simulink model "mode06_net"  (Simulink 7.4)
settings: Solver=ode45  StartTime=0.0  StopTime=5200  RelTol=1e-3
undefined symbols (not defined in the file or in its folder): ROACH
libraries: xbsIndex_r4 x184, xps_library x20, casper_library_misc x19, dspsigops x16, casper_library_flow_control x2
(part 2 of 2)

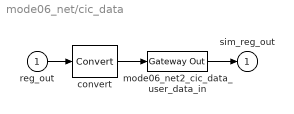
== system mode06_net/cic_data ==
  reg_out : Inport
  convert : xbsIndex_r4/Convert  arith_type=Unsigned  n_bits=32  bin_pt=0  quantization=Truncate  overflow=Wrap  latency=0  dbl_ovrd=off  pipeline=off  block_type=convert
      settings: block_version=11.4
  mode06_net2_cic_data_user_data_in : xbsIndex_r4/Gateway Out  hdl_port=on  timing_constraint=None  locs_specified=off  LOCs={}  block_type=gatewayout
      settings: infoedit="Gateway out block.  Converts Xilinx fixed point inputs into ouputs of type Simulink integer, double, or fixed point.<br><br>Hardware notes:  In hardware these blocks become top level output ports or are discarded, depending on how they are configured."  block_version=11.4
  sim_reg_out : Outport
  wires:
  mode06_net2_cic_data_user_data_in/1 -> sim_reg_out/1
  convert/1 -> mode06_net2_cic_data_user_data_in/1
  reg_out/1 -> convert/1

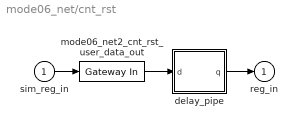
== system mode06_net/cnt_rst ==
  sim_reg_in : Inport
  delay_pipe : Subsystem
  mode06_net2_cnt_rst_user_data_out : xbsIndex_r4/Gateway In  arith_type=Unsigned  n_bits=32  bin_pt=0  quantization="Round  (unbiased: +/- Inf)"  overflow=Saturate  period=1  dbl_ovrd=off  timing_constraint=None  locs_specified=off  LOCs={}  hdl_port=on  block_type=gatewayin
      settings: infoedit="Gateway in block.  Converts inputs of type Simulink integer, double and fixed point to  Xilinx fixed point type.<br><br>Hardware notes:  In hardware these blocks become top level input ports."  block_version=11.4
  reg_in : Outport
  wires:
  delay_pipe/1(q) -> reg_in/1
  mode06_net2_cnt_rst_user_data_out/1 -> delay_pipe/1(d)
  sim_reg_in/1 -> mode06_net2_cnt_rst_user_data_out/1

== system mode06_net/dest_ip ==
  sim_reg_in : Inport
  delay_pipe : Subsystem
  mode06_net2_dest_ip_user_data_out : xbsIndex_r4/Gateway In  arith_type=Unsigned  n_bits=32  bin_pt=0  quantization="Round  (unbiased: +/- Inf)"  overflow=Saturate  period=1  dbl_ovrd=off  timing_constraint=None  locs_specified=off  LOCs={}  hdl_port=on  block_type=gatewayin
      settings: infoedit="Gateway in block.  Converts inputs of type Simulink integer, double and fixed point to  Xilinx fixed point type.<br><br>Hardware notes:  In hardware these blocks become top level input ports."  block_version=11.4
  reg_in : Outport
  wires:
  delay_pipe/1(q) -> reg_in/1
  mode06_net2_dest_ip_user_data_out/1 -> delay_pipe/1(d)
  sim_reg_in/1 -> mode06_net2_dest_ip_user_data_out/1

== system mode06_net/dest_port ==
  sim_reg_in : Inport
  delay_pipe : Subsystem
  mode06_net2_dest_port_user_data_out : xbsIndex_r4/Gateway In  arith_type=Unsigned  n_bits=32  bin_pt=0  quantization="Round  (unbiased: +/- Inf)"  overflow=Saturate  period=1  dbl_ovrd=off  timing_constraint=None  locs_specified=off  LOCs={}  hdl_port=on  block_type=gatewayin
      settings: infoedit="Gateway in block.  Converts inputs of type Simulink integer, double and fixed point to  Xilinx fixed point type.<br><br>Hardware notes:  In hardware these blocks become top level input ports."  block_version=11.4
  reg_in : Outport
  wires:
  delay_pipe/1(q) -> reg_in/1
  mode06_net2_dest_port_user_data_out/1 -> delay_pipe/1(d)
  sim_reg_in/1 -> mode06_net2_dest_port_user_data_out/1

== system mode06_net/eth_rst ==
  sim_reg_in : Inport
  delay_pipe : Subsystem
  mode06_net2_eth_rst_user_data_out : xbsIndex_r4/Gateway In  arith_type=Unsigned  n_bits=32  bin_pt=0  quantization="Round  (unbiased: +/- Inf)"  overflow=Saturate  period=1  dbl_ovrd=off  timing_constraint=None  locs_specified=off  LOCs={}  hdl_port=on  block_type=gatewayin
      settings: infoedit="Gateway in block.  Converts inputs of type Simulink integer, double and fixed point to  Xilinx fixed point type.<br><br>Hardware notes:  In hardware these blocks become top level input ports."  block_version=11.4
  reg_in : Outport
  wires:
  delay_pipe/1(q) -> reg_in/1
  mode06_net2_eth_rst_user_data_out/1 -> delay_pipe/1(d)
  sim_reg_in/1 -> mode06_net2_eth_rst_user_data_out/1

== system mode06_net/ext_sync_ctr ==
  reg_out : Inport
  convert : xbsIndex_r4/Convert  arith_type=Unsigned  n_bits=32  bin_pt=0  quantization=Truncate  overflow=Wrap  latency=0  dbl_ovrd=off  pipeline=off  block_type=convert
      settings: block_version=11.4
  mode06_net2_ext_sync_ctr_user_data_in : xbsIndex_r4/Gateway Out  hdl_port=on  timing_constraint=None  locs_specified=off  LOCs={}  block_type=gatewayout
      settings: infoedit="Gateway out block.  Converts Xilinx fixed point inputs into ouputs of type Simulink integer, double, or fixed point.<br><br>Hardware notes:  In hardware these blocks become top level output ports or are discarded, depending on how they are configured."  block_version=11.4
  sim_reg_out : Outport
  wires:
  mode06_net2_ext_sync_ctr_user_data_in/1 -> sim_reg_out/1
  convert/1 -> mode06_net2_ext_sync_ctr_user_data_in/1
  reg_out/1 -> convert/1

== system mode06_net/ip_select ==
  sim_reg_in : Inport
  delay_pipe : Subsystem
  mode06_net2_ip_select_user_data_out : xbsIndex_r4/Gateway In  arith_type=Unsigned  n_bits=32  bin_pt=0  quantization="Round  (unbiased: +/- Inf)"  overflow=Saturate  period=1  dbl_ovrd=off  timing_constraint=None  locs_specified=off  LOCs={}  hdl_port=on  block_type=gatewayin
      settings: infoedit="Gateway in block.  Converts inputs of type Simulink integer, double and fixed point to  Xilinx fixed point type.<br><br>Hardware notes:  In hardware these blocks become top level input ports."  block_version=11.4
  reg_in : Outport
  wires:
  delay_pipe/1(q) -> reg_in/1
  mode06_net2_ip_select_user_data_out/1 -> delay_pipe/1(d)
  sim_reg_in/1 -> mode06_net2_ip_select_user_data_out/1

== system mode06_net/pkt_data ==
  reg_out : Inport
  convert : xbsIndex_r4/Convert  arith_type=Unsigned  n_bits=32  bin_pt=0  quantization=Truncate  overflow=Wrap  latency=0  dbl_ovrd=off  pipeline=off  block_type=convert
      settings: block_version=11.4
  mode06_net2_pkt_data_user_data_in : xbsIndex_r4/Gateway Out  hdl_port=on  timing_constraint=None  locs_specified=off  LOCs={}  block_type=gatewayout
      settings: infoedit="Gateway out block.  Converts Xilinx fixed point inputs into ouputs of type Simulink integer, double, or fixed point.<br><br>Hardware notes:  In hardware these blocks become top level output ports or are discarded, depending on how they are configured."  block_version=11.4
  sim_reg_out : Outport
  wires:
  mode06_net2_pkt_data_user_data_in/1 -> sim_reg_out/1
  convert/1 -> mode06_net2_pkt_data_user_data_in/1
  reg_out/1 -> convert/1

== system mode06_net/port_select ==
  sim_reg_in : Inport
  delay_pipe : Subsystem
  mode06_net2_port_select_user_data_out : xbsIndex_r4/Gateway In  arith_type=Unsigned  n_bits=32  bin_pt=0  quantization="Round  (unbiased: +/- Inf)"  overflow=Saturate  period=1  dbl_ovrd=off  timing_constraint=None  locs_specified=off  LOCs={}  hdl_port=on  block_type=gatewayin
      settings: infoedit="Gateway in block.  Converts inputs of type Simulink integer, double and fixed point to  Xilinx fixed point type.<br><br>Hardware notes:  In hardware these blocks become top level input ports."  block_version=11.4
  reg_in : Outport
  wires:
  delay_pipe/1(q) -> reg_in/1
  mode06_net2_port_select_user_data_out/1 -> delay_pipe/1(d)
  sim_reg_in/1 -> mode06_net2_port_select_user_data_out/1

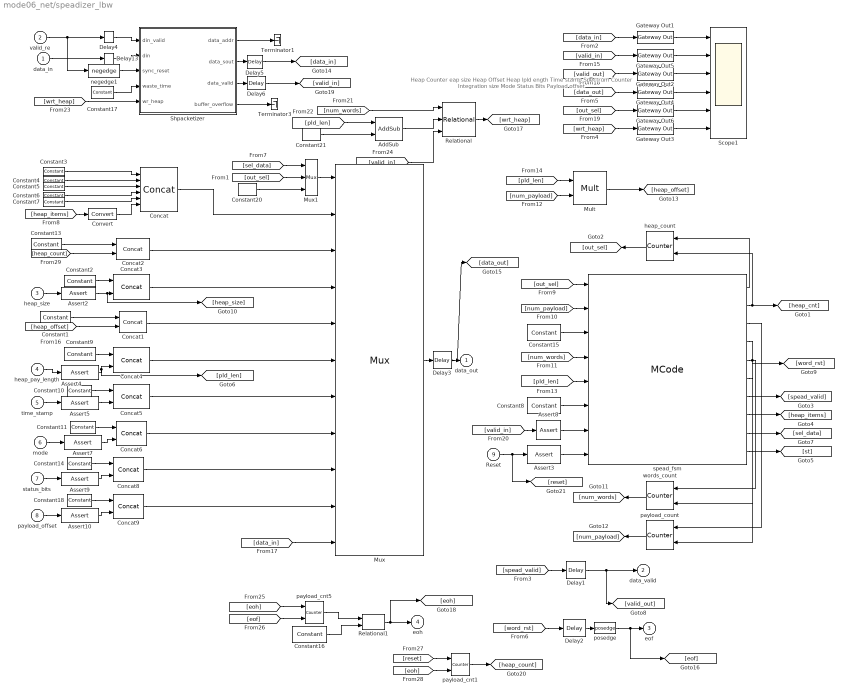
== system mode06_net/speadizer_lbw ==
  note: Heap Counter
      | eap size
      | Heap Offset
      | Heap lpld ength
      | Time stamp
      | Spectrum Counter
      | Integration size
      | Mode
      | Status Bits
      | Payload offset
  data_in : Inport
  valid_re : Inport  Port=2
  heap_size : Inport  Port=3
  heap_pay_length : Inport  Port=4
  time_stamp : Inport  Port=5
  mode : Inport  Port=6
  status_bits : Inport  Port=7
  payload_offset : Inport  Port=8
  Reset : Inport  Port=9
  AddSub : xbsIndex_r4/AddSub  mode=Subtraction  use_carryin=off  use_carryout=off  en=off  latency=0  precision=Full  arith_type=Unsigned  n_bits=16  bin_pt=14  quantization=Truncate  overflow=Wrap  dbl_ovrd=off  use_behavioral_HDL=off  hw_selection=Fabric  pipelined=off  block_type=addsub
  Assert{2,4..5,7,9..10} (6 alike) : xbsIndex_r4/Assert  assert_type=on  type_source=Explicitly  arith_type=Unsigned  n_bits=spead_lsw  bin_pt=0  assert_rate=off  rate_source=Explicitly  period=1  output_port=on  block_type=assert
      settings: block_version=11.4
  Assert3 : xbsIndex_r4/Assert  assert_type=on  type_source=Explicitly  arith_type=Boolean  n_bits=spead_lsw  bin_pt=0  assert_rate=on  rate_source=Explicitly  period=1  output_port=on  block_type=assert
      settings: block_version=11.4
  Assert8 : xbsIndex_r4/Assert  assert_type=on  type_source=Explicitly  arith_type=Boolean  n_bits=spead_lsw  bin_pt=0  assert_rate=on  rate_source=Explicitly  period=1  output_port=on  block_type=assert
      settings: block_version=11.4
  Concat : xbsIndex_r4/Concat  num_inputs=6  dbl_ovrd=off  block_type=concat
  Concat{1..6,8..9} (8 alike) : xbsIndex_r4/Concat  num_inputs=2  dbl_ovrd=off  block_type=concat
  Constant1 : xbsIndex_r4/Constant  arith_type=Unsigned  const=8388608+3  n_bits=spead_msw-spead_lsw  bin_pt=0  explicit_period=on  period=1  equ=P=C  opselect=C  inp2=PCIN>>17  opr=+  inp1=P  carry=CIN  dbl_ovrd=off  block_type=constant
      settings: block_version=11.4
  Constant10 : xbsIndex_r4/Constant  arith_type=Unsigned  const=8388608+32  n_bits=spead_msw-spead_lsw  bin_pt=0  explicit_period=on  period=1  equ=P=C  opselect=C  inp2=PCIN>>17  opr=+  inp1=P  carry=CIN  dbl_ovrd=off  block_type=constant
      settings: block_version=11.4
  Constant11 : xbsIndex_r4/Constant  arith_type=Unsigned  const=8388608+33  n_bits=spead_msw-spead_lsw  bin_pt=0  explicit_period=on  period=1  equ=P=C  opselect=C  inp2=PCIN>>17  opr=+  inp1=P  carry=CIN  dbl_ovrd=off  block_type=constant
      settings: block_version=11.4
  Constant13 : xbsIndex_r4/Constant  arith_type=Unsigned  const=8388608+1  n_bits=spead_msw-spead_lsw  bin_pt=0  explicit_period=on  period=1  equ=P=C  opselect=C  inp2=PCIN>>17  opr=+  inp1=P  carry=CIN  dbl_ovrd=off  block_type=constant
      settings: block_version=11.4
  Constant14 : xbsIndex_r4/Constant  arith_type=Unsigned  const=8388608+34  n_bits=spead_msw-spead_lsw  bin_pt=0  explicit_period=on  period=1  equ=P=C  opselect=C  inp2=PCIN>>17  opr=+  inp1=P  carry=CIN  dbl_ovrd=off  block_type=constant
      settings: block_version=11.4
  Constant15 : xbsIndex_r4/Constant  arith_type=Unsigned  const=num_items+5  n_bits=8  bin_pt=0  explicit_period=on  period=1  equ=P=C  opselect=C  inp2=PCIN>>17  opr=+  inp1=P  carry=CIN  dbl_ovrd=off  block_type=constant
      settings: block_version=11.4
  Constant16 : xbsIndex_r4/Constant  arith_type=Unsigned  const=num_payloads  n_bits=4  bin_pt=0  explicit_period=on  period=1  equ=P=C  opselect=C  inp2=PCIN>>17  opr=+  inp1=P  carry=CIN  dbl_ovrd=off  block_type=constant
      settings: block_version=11.4
  Constant17 : xbsIndex_r4/Constant  arith_type=Unsigned  const=7  n_bits=7  bin_pt=0  explicit_period=on  period=1  equ=P=C  opselect=C  inp2=PCIN>>17  opr=+  inp1=P  carry=CIN  dbl_ovrd=off  block_type=constant
  Constant18 : xbsIndex_r4/Constant  arith_type=Unsigned  const=0+35  n_bits=spead_msw-spead_lsw  bin_pt=0  explicit_period=on  period=1  equ=P=C  opselect=C  inp2=PCIN>>17  opr=+  inp1=P  carry=CIN  dbl_ovrd=off  block_type=constant
      settings: block_version=11.4
  Constant2 : xbsIndex_r4/Constant  arith_type=Unsigned  const=8388608+2  n_bits=spead_msw-spead_lsw  bin_pt=0  explicit_period=on  period=1  equ=P=C  opselect=C  inp2=PCIN>>17  opr=+  inp1=P  carry=CIN  dbl_ovrd=off  block_type=constant
      settings: block_version=11.4
  Constant20 : xbsIndex_r4/Constant  arith_type=Unsigned  const=num_items+5  n_bits=4  bin_pt=0  explicit_period=on  period=1  equ=P=C  opselect=C  inp2=PCIN>>17  opr=+  inp1=P  carry=CIN  dbl_ovrd=off  block_type=constant
      settings: block_version=11.4
  Constant21 : xbsIndex_r4/Constant  arith_type=Unsigned  const=16  n_bits=5  bin_pt=0  explicit_period=on  period=1  equ=P=C  opselect=C  inp2=PCIN>>17  opr=+  inp1=P  carry=CIN  dbl_ovrd=off  block_type=constant
      settings: block_version=11.4
  Constant3 : xbsIndex_r4/Constant  arith_type=Unsigned  const=83  n_bits=8  bin_pt=0  explicit_period=on  period=1  equ=P=C  opselect=C  inp2=PCIN>>17  opr=+  inp1=P  carry=CIN  dbl_ovrd=off  block_type=constant
      settings: block_version=11.4
  Constant4 : xbsIndex_r4/Constant  arith_type=Unsigned  const=4  n_bits=8  bin_pt=0  explicit_period=on  period=1  equ=P=C  opselect=C  inp2=PCIN>>17  opr=+  inp1=P  carry=CIN  dbl_ovrd=off  block_type=constant
      settings: block_version=11.4
  Constant5 : xbsIndex_r4/Constant  arith_type=Unsigned  const=3  n_bits=8  bin_pt=0  explicit_period=on  period=1  equ=P=C  opselect=C  inp2=PCIN>>17  opr=+  inp1=P  carry=CIN  dbl_ovrd=off  block_type=constant
      settings: block_version=11.4
  Constant6 : xbsIndex_r4/Constant  arith_type=Unsigned  const=5  n_bits=8  bin_pt=0  explicit_period=on  period=1  equ=P=C  opselect=C  inp2=PCIN>>17  opr=+  inp1=P  carry=CIN  dbl_ovrd=off  block_type=constant
      settings: block_version=11.4
  Constant7 : xbsIndex_r4/Constant  arith_type=Unsigned  const=0  n_bits=16  bin_pt=0  explicit_period=on  period=1  equ=P=C  opselect=C  inp2=PCIN>>17  opr=+  inp1=P  carry=CIN  dbl_ovrd=off  block_type=constant
      settings: block_version=11.4
  Constant8 : xbsIndex_r4/Constant  arith_type=Unsigned  const=num_payloads  n_bits=8  bin_pt=0  explicit_period=on  period=1  equ=P=C  opselect=C  inp2=PCIN>>17  opr=+  inp1=P  carry=CIN  dbl_ovrd=off  block_type=constant
      settings: block_version=11.4
  Constant9 : xbsIndex_r4/Constant  arith_type=Unsigned  const=8388608+4  n_bits=spead_msw-spead_lsw  bin_pt=0  explicit_period=on  period=1  equ=P=C  opselect=C  inp2=PCIN>>17  opr=+  inp1=P  carry=CIN  dbl_ovrd=off  block_type=constant
      settings: block_version=11.4
  Convert : xbsIndex_r4/Convert  arith_type=Unsigned  n_bits=16  bin_pt=0  quantization=Truncate  overflow=Wrap  latency=0  dbl_ovrd=off  pipeline=off  block_type=convert
      settings: block_version=11.4
  Delay1 : xbsIndex_r4/Delay  en=off  latency=1  dbl_ovrd=off  reg_retiming=on  block_type=delay
      settings: block_version=11.4
  Delay13 : xbsIndex_r4/Delay  en=off  latency=2  dbl_ovrd=off  reg_retiming=off  block_type=delay
      settings: block_version=11.4
  Delay2 : xbsIndex_r4/Delay  en=off  latency=0  dbl_ovrd=off  reg_retiming=on  block_type=delay
      settings: block_version=11.4
  Delay3 : xbsIndex_r4/Delay  en=off  latency=1  dbl_ovrd=off  reg_retiming=on  block_type=delay
      settings: block_version=11.4
  Delay4 : xbsIndex_r4/Delay  en=off  latency=2  dbl_ovrd=off  reg_retiming=off  block_type=delay
      settings: block_version=11.4
  Delay5 : xbsIndex_r4/Delay  en=off  latency=3  dbl_ovrd=off  reg_retiming=on  block_type=delay
      settings: block_version=11.4
  Delay6 : xbsIndex_r4/Delay  en=off  latency=3  dbl_ovrd=off  reg_retiming=on  block_type=delay
      settings: block_version=11.4
  Gateway Out{1..6} (6 alike) : xbsIndex_r4/Gateway Out  hdl_port=on  timing_constraint=None  locs_specified=off  LOCs={}  block_type=gatewayout
      settings: infoedit="Gateway out block.  Converts Xilinx fixed point inputs into ouputs of type Simulink integer, double, or fixed point.<br><br>Hardware notes:  In hardware these blocks become top level output ports or are discarded, depending on how they are configured."  block_version=11.4
  Mult : xbsIndex_r4/Mult  precision=User Defined  arith_type=Unsigned  n_bits=40  bin_pt=0  quantization=Truncate  overflow=Wrap  en=off  latency=3  dbl_ovrd=off  use_behavioral_HDL=off  opt=Speed  use_embedded=on  optimum_pipeline=off  pipeline=on  use_rpm=on  placement_style=Triangular  block_type=mult
      settings: block_version=11.4
  Mux : xbsIndex_r4/Mux  inputs=10  en=off  latency=0  precision=User Defined  arith_type=Unsigned  n_bits=64  bin_pt=0  quantization=Truncate  overflow=Wrap  dbl_ovrd=off  block_type=mux
      settings: block_version=11.4
  Mux1 : xbsIndex_r4/Mux  inputs=2  en=off  latency=0  precision=Full  arith_type="Signed  (2's comp)"  n_bits=8  bin_pt=2  quantization=Truncate  overflow=Wrap  dbl_ovrd=off  block_type=mux
      settings: block_version=11.4
  Relational : xbsIndex_r4/Relational  mode=a>=b  en=on  latency=1  dbl_ovrd=off  block_type=relational
  Relational1 : xbsIndex_r4/Relational  mode=a=b  en=off  latency=0  dbl_ovrd=off  block_type=relational
  Scope1 : Scope  NumInputPorts=6
      settings: TimeRange=1000  YMin=0~0~0~0~0~0  YMax=40~1~1~1e+19~1~20  SaveName=ScopeData2  MaxDataPoints=10000
  Shpacketizer : Subsystem  AncestorBlock=gbt_library/Spacketizer  mask(shpacketizer){pin_width=128, sout_width=64, fifo_depth=128, total_words=2048}
      mask prompts: pin_width "Parallel Input Width"; sout_width "Serial Output Width"; fifo_depth "FIFO depth"; total_words "Total number of data points"
      mask help:
      | This block is intended to serialize data that is 'bursty', that is,
      | the average data rate is small but per cycle the data is highly
      | parallel and can contain many points simultaneously.  This situation
      | is common with the streaming CASPER FFTs and related blocks.
      |
      | The serialization buffers the data when valid and independently
      | serializes the data when the buffer is non-empty.  For convenience, the
      | data is counted as it is serialized and signals exist to indicate
      | that the serial output is valid or that a buffer overflow has occured.  The
      | block will not stop in the case of an overflow, and the overflow
      | signal is not held high after it occurs.
      |
      | For example usage, see 'roach_spec_2adc_borph' in 'SVNROOT/trunk/projects/roach_spec/'
      | or the test case in 'SVNROOT/trunk/mlib_devel_10_1/Tests/packetizer_test.mdl'
      |
      | For extended documentation, please see the CASPER wiki
      mask init:
      | shpacketizer_init(gcb, 'pin_width', pin_width, 'sout_width', sout_width, 'total_words', total_words, 'fifo_depth', fifo_depth)
      | % packetizer_init(gcb, ...
      | %     'pin_width', pin_width, ...
      | %     'sout_width', sout_width, ...
      | %   %  'fifo_depth', fifo_depth, ...
      | %     'total_words', total_words);
      settings: AttributesFormatString=|
      | Parallel Input Width: 128
      | Serial Output Width: 64
      mask StyleString: edit,edit,popup(16|32|64|128|256|512|1K|2K|4K|8K|16K|32K|64K),edit
  Terminator1 : Terminator
  Terminator3 : Terminator
  heap_count : xbsIndex_r4/Counter  cnt_type=Free Running  cnt_to=Inf  operation=Up  start_count=0  cnt_by_val=1  arith_type=Unsigned  n_bits=4  bin_pt=0  load_pin=off  rst=on  en=on  explicit_period=on  period=1  dbl_ovrd=off  use_behavioral_HDL=off  implementation=Fabric  block_type=counter
      settings: block_version=11.4
  negedge1 : casper_library_misc/negedge  Tag=Rising Edge Detector  SystemSampleTime=-1
  payload_cnt1 : xbsIndex_r4/Counter  cnt_type=Free Running  cnt_to=0  operation=Up  start_count=1024  cnt_by_val=1  arith_type=Unsigned  n_bits=40  bin_pt=0  load_pin=off  rst=on  en=on  explicit_period=on  period=1  dbl_ovrd=off  use_behavioral_HDL=off  implementation=Fabric  use_rpm=on  block_type=counter
      settings: xl_area=[0, 0, 0, 0, 0, 0, 0]
  payload_cnt5 : xbsIndex_r4/Counter  cnt_type=Free Running  cnt_to=0  operation=Up  start_count=0  cnt_by_val=1  arith_type=Unsigned  n_bits=4  bin_pt=0  load_pin=off  rst=on  en=on  explicit_period=on  period=1  dbl_ovrd=off  use_behavioral_HDL=off  implementation=Fabric  use_rpm=on  block_type=counter
      settings: xl_area=[0, 0, 0, 0, 0, 0, 0]
  payload_count : xbsIndex_r4/Counter  cnt_type=Free Running  cnt_to=Inf  operation=Up  start_count=0  cnt_by_val=1  arith_type=Unsigned  n_bits=8  bin_pt=0  load_pin=off  rst=on  en=on  explicit_period=on  period=1  dbl_ovrd=off  use_behavioral_HDL=off  implementation=Fabric  block_type=counter
      settings: block_version=11.4
  posedge : casper_library_misc/posedge  Tag=Rising Edge Detector  SystemSampleTime=-1
  spead_fsm : xbsIndex_r4/MCode  mfname=spead_fsm  explicit_period=on  period=1  inputsTable={'boundInpExpr'=>['','','','5','','','','',''],'inputs'=>['head_count','num_payload_sent','total_header_len','min_header_len','num_words_sent','payload_len','total_num_payloads','data_valid_in','rst']}  outputsTable={'outputs'=>['head_count_rst','head_count_en','num_payload_rst','num_payload_en','words_sent_rst','words_sent_en','tge_valid','heap_elements','select_data','st'],'suppressOut'=>['off','off','off','off','off','off','off','off','off','off']}  dbl_ovrd=off  enable_stdout=off  enable_debug=off  suppress_output=on  defparams={'min_header_len',5}  hide_port_list={}  block_type=mcode
      settings: block_version=11.4
  words_count : xbsIndex_r4/Counter  cnt_type=Free Running  cnt_to=Inf  operation=Up  start_count=0  cnt_by_val=8  arith_type=Unsigned  n_bits=15  bin_pt=0  load_pin=off  rst=on  en=on  explicit_period=on  period=1  dbl_ovrd=off  use_behavioral_HDL=off  implementation=Fabric  block_type=counter
      settings: block_version=11.4
  data_out : Outport
  data_valid : Outport  Port=2
  eof : Outport  Port=3
  eoh : Outport  Port=4
  wires:
  Assert10/1 -> Concat9/2
  Constant18/1 -> Concat9/1
  Concat4/1 -> Mux/6
  Concat3/1 -> Mux/4
  Concat/1 -> Mux/2
  Constant9/1 -> Concat4/1
  Constant7/1 -> Concat/5
  Constant6/1 -> Concat/4
  Constant5/1 -> Concat/3
  Constant4/1 -> Concat/2
  Constant3/1 -> Concat/1
  Constant2/1 -> Concat3/1
  Constant10/1 -> Concat5/1
  time_stamp/1 -> Assert5/1
  heap_size/1 -> Assert2/1
  Assert2/1 -> Concat3/2, [heap_size]
  Assert4/1 -> Concat4/2, [pld_len]
  Assert5/1 -> Concat5/2
  [spead_valid] -> Delay1/1
  heap_pay_length/1 -> Assert4/1
  [valid_out] -> Gateway Out2/1
  Delay1/1 -> data_valid/1, [valid_out]
  [out_sel] -> Gateway Out6/1
  Constant1/1 -> Concat1/1
  Concat1/1 -> Mux/5
  Concat9/1 -> Mux/10
  Assert7/1 -> Concat6/2
  Constant11/1 -> Concat6/1
  Concat6/1 -> Mux/8
  Concat5/1 -> Mux/7
  Assert9/1 -> Concat8/2
  Constant14/1 -> Concat8/1
  Concat8/1 -> Mux/9
  Gateway Out2/1 -> Scope1/3
  Gateway Out6/1 -> Scope1/5
  spead_fsm/5 -> words_count/1
  spead_fsm/6 -> words_count/2
  spead_fsm/3 -> payload_count/1
  spead_fsm/4 -> payload_count/2, [word_rst]
  spead_fsm/1 -> heap_count/1
  spead_fsm/2 -> heap_count/2, [heap_cnt]
  spead_fsm/7 -> [spead_valid]
  spead_fsm/8 -> [heap_items]
  [heap_offset] -> Concat1/2
  Reset/1 -> Assert3/1, [reset]
  [data_in] -> Gateway Out1/1
  Gateway Out1/1 -> Scope1/1
  Gateway Out3/1 -> Scope1/6
  Gateway Out4/1 -> Scope1/4
  [data_out] -> Gateway Out4/1
  Constant20/1 -> Mux1/3
  Mux1/1 -> Mux/1
  spead_fsm/10 -> [st]
  spead_fsm/9 -> [sel_data]
  [heap_items] -> Convert/1
  Convert/1 -> Concat/6
  words_count/1 -> [num_words]
  payload_count/1 -> [num_payload]
  heap_count/1 -> [out_sel]
  [out_sel] -> spead_fsm/1
  [num_payload] -> spead_fsm/2
  [valid_in] -> Gateway Out5/1
  Gateway Out5/1 -> Scope1/2
  posedge/1 -> eof/1, [eof]
  [word_rst] -> Delay2/1
  Assert3/1 -> spead_fsm/8
  Assert8/1 -> spead_fsm/7
  Constant8/1 -> spead_fsm/6
  [pld_len] -> spead_fsm/5
  [num_words] -> spead_fsm/4
  Constant15/1 -> spead_fsm/3
  Delay2/1 -> posedge/1
  [num_payload] -> Mult/2
  [pld_len] -> Mult/1
  Mult/1 -> [heap_offset]
  Delay3/1 -> data_out/1, [data_out]
  Mux/1 -> Delay3/1
  [out_sel] -> Mux1/2
  [sel_data] -> Mux1/1
  [wrt_heap] -> Gateway Out3/1
  Shpacketizer/2(data_sout) -> Delay5/1
  data_in/1 -> Delay13/1
  Shpacketizer/4(buffer_overflow) -> Terminator3/1
  Shpacketizer/1(data_addr) -> Terminator1/1
  Delay5/1 -> [data_in]
  Shpacketizer/3(data_valid) -> Delay6/1
  Delay6/1 -> [valid_in]
  [valid_in] -> Assert8/1
  valid_re/1 -> Delay4/1, negedge1/1
  Delay4/1 -> Shpacketizer/1(din_valid)
  Constant17/1 -> Shpacketizer/4(waste_time)
  negedge1/1 -> Shpacketizer/3(sync_reset)
  Delay13/1 -> Shpacketizer/2(din)
  [wrt_heap] -> Shpacketizer/5(wr_heap)
  [num_words] -> Relational/1
  [pld_len] -> AddSub/1
  Constant21/1 -> AddSub/2
  AddSub/1 -> Relational/2
  Relational/1 -> [wrt_heap]
  [valid_in] -> Relational/3
  [eoh] -> payload_cnt5/1
  [eof] -> payload_cnt5/2
  Relational1/1 -> eoh/1, [eoh]
  Constant16/1 -> Relational1/2
  payload_cnt5/1 -> Relational1/1
  payload_cnt1/1 -> [heap_count]
  [reset] -> payload_cnt1/1
  [eoh] -> payload_cnt1/2
  Constant13/1 -> Concat2/1
  [heap_count] -> Concat2/2
  Concat2/1 -> Mux/3
  mode/1 -> Assert7/1
  status_bits/1 -> Assert9/1
  payload_offset/1 -> Assert10/1
  [data_in] -> Mux/11

== system mode06_net/sync_en ==
  sim_reg_in : Inport
  delay_pipe : Subsystem
  mode06_net2_sync_en_user_data_out : xbsIndex_r4/Gateway In  arith_type=Unsigned  n_bits=32  bin_pt=0  quantization="Round  (unbiased: +/- Inf)"  overflow=Saturate  period=1  dbl_ovrd=off  timing_constraint=None  locs_specified=off  LOCs={}  hdl_port=on  block_type=gatewayin
      settings: infoedit="Gateway in block.  Converts inputs of type Simulink integer, double and fixed point to  Xilinx fixed point type.<br><br>Hardware notes:  In hardware these blocks become top level input ports."  block_version=11.4
  reg_in : Outport
  wires:
  delay_pipe/1(q) -> reg_in/1
  mode06_net2_sync_en_user_data_out/1 -> delay_pipe/1(d)
  sim_reg_in/1 -> mode06_net2_sync_en_user_data_out/1

== system mode06_net/sync_period ==
  sim_reg_in : Inport
  delay_pipe : Subsystem
  mode06_net2_sync_period_user_data_out : xbsIndex_r4/Gateway In  arith_type=Unsigned  n_bits=32  bin_pt=0  quantization="Round  (unbiased: +/- Inf)"  overflow=Saturate  period=1  dbl_ovrd=off  timing_constraint=None  locs_specified=off  LOCs={}  hdl_port=on  block_type=gatewayin
      settings: infoedit="Gateway in block.  Converts inputs of type Simulink integer, double and fixed point to  Xilinx fixed point type.<br><br>Hardware notes:  In hardware these blocks become top level input ports."  block_version=11.4
  reg_in : Outport
  wires:
  delay_pipe/1(q) -> reg_in/1
  mode06_net2_sync_period_user_data_out/1 -> delay_pipe/1(d)
  sim_reg_in/1 -> mode06_net2_sync_period_user_data_out/1

== system mode06_net/sync_sel ==
  sim_reg_in : Inport
  delay_pipe : Subsystem
  mode06_net2_sync_sel_user_data_out : xbsIndex_r4/Gateway In  arith_type=Unsigned  n_bits=32  bin_pt=0  quantization="Round  (unbiased: +/- Inf)"  overflow=Saturate  period=1  dbl_ovrd=off  timing_constraint=None  locs_specified=off  LOCs={}  hdl_port=on  block_type=gatewayin
      settings: infoedit="Gateway in block.  Converts inputs of type Simulink integer, double and fixed point to  Xilinx fixed point type.<br><br>Hardware notes:  In hardware these blocks become top level input ports."  block_version=11.4
  reg_in : Outport
  wires:
  delay_pipe/1(q) -> reg_in/1
  mode06_net2_sync_sel_user_data_out/1 -> delay_pipe/1(d)
  sim_reg_in/1 -> mode06_net2_sync_sel_user_data_out/1

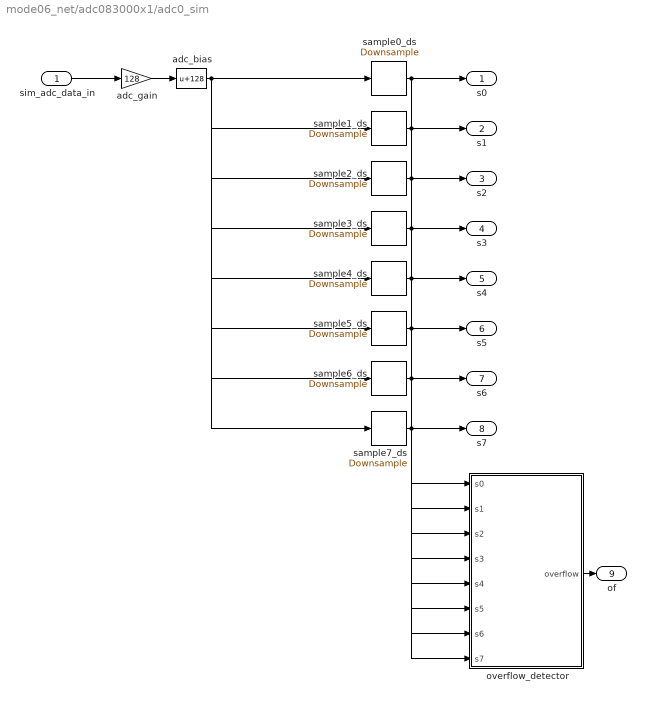
== system mode06_net/adc083000x1/adc0_sim ==
  sim_adc_data_in : Inport  OutDataType=sfix(16)  OutScaling=2^0
  adc_bias : Bias  Bias=128  SaturateOnIntegerOverflow=on
  adc_gain : Gain  Gain=128  ParameterDataType=sfix(16)  ParameterScaling=2^0  OutDataType=sfix(16)  OutScaling=2^0
  overflow_detector : Subsystem  AncestorBlock=casper_library/Misc/of_detect_bus  mask(of_detect_bus){nStreams=8, bit_width=8}
      mask prompts: nStreams "Number of Streams"; bit_width "Bit Width"
      mask init:
      | adc_overflow_detector_init(gcb, ...
      |     'nStreams', nStreams, ...
      |     'bit_width', bit_width);
  sample0_ds : dspsigops/Downsample  N=8  phase=1  ic=0  smode=Force single rate  fmode=Maintain input frame size
  sample1_ds : dspsigops/Downsample  N=8  phase=2  ic=0  smode=Force single rate  fmode=Maintain input frame size
  sample2_ds : dspsigops/Downsample  N=8  phase=3  ic=0  smode=Force single rate  fmode=Maintain input frame size
  sample3_ds : dspsigops/Downsample  N=8  phase=4  ic=0  smode=Force single rate  fmode=Maintain input frame size
  sample4_ds : dspsigops/Downsample  N=8  phase=5  ic=0  smode=Force single rate  fmode=Maintain input frame size
  sample5_ds : dspsigops/Downsample  N=8  phase=6  ic=0  smode=Force single rate  fmode=Maintain input frame size
  sample6_ds : dspsigops/Downsample  N=8  phase=7  ic=0  smode=Force single rate  fmode=Maintain input frame size
  sample7_ds : dspsigops/Downsample  N=8  phase=0  ic=0  smode=Force single rate  fmode=Maintain input frame size
  s0 : Outport  OutDataType=sfix(16)  OutScaling=2^0
  s1 : Outport  Port=2  OutDataType=sfix(16)  OutScaling=2^0
  s2 : Outport  Port=3  OutDataType=sfix(16)  OutScaling=2^0
  s3 : Outport  Port=4  OutDataType=sfix(16)  OutScaling=2^0
  s4 : Outport  Port=5  OutDataType=sfix(16)  OutScaling=2^0
  s5 : Outport  Port=6  OutDataType=sfix(16)  OutScaling=2^0
  s6 : Outport  Port=7  OutDataType=sfix(16)  OutScaling=2^0
  s7 : Outport  Port=8  OutDataType=sfix(16)  OutScaling=2^0
  of : Outport  Port=9  OutDataType=sfix(16)  OutScaling=2^0
  wires:
  sim_adc_data_in/1 -> adc_gain/1
  adc_gain/1 -> adc_bias/1
  overflow_detector/1(overflow) -> of/1
  adc_bias/1 -> sample0_ds/1, sample1_ds/1, sample2_ds/1, sample3_ds/1, sample4_ds/1, sample5_ds/1, sample6_ds/1, sample7_ds/1
  sample0_ds/1 -> overflow_detector/1(s0), s0/1
  sample1_ds/1 -> overflow_detector/2(s1), s1/1
  sample2_ds/1 -> overflow_detector/3(s2), s2/1
  sample3_ds/1 -> overflow_detector/4(s3), s3/1
  sample4_ds/1 -> overflow_detector/5(s4), s4/1
  sample5_ds/1 -> overflow_detector/6(s5), s5/1
  sample6_ds/1 -> overflow_detector/7(s6), s6/1
  sample7_ds/1 -> overflow_detector/8(s7), s7/1

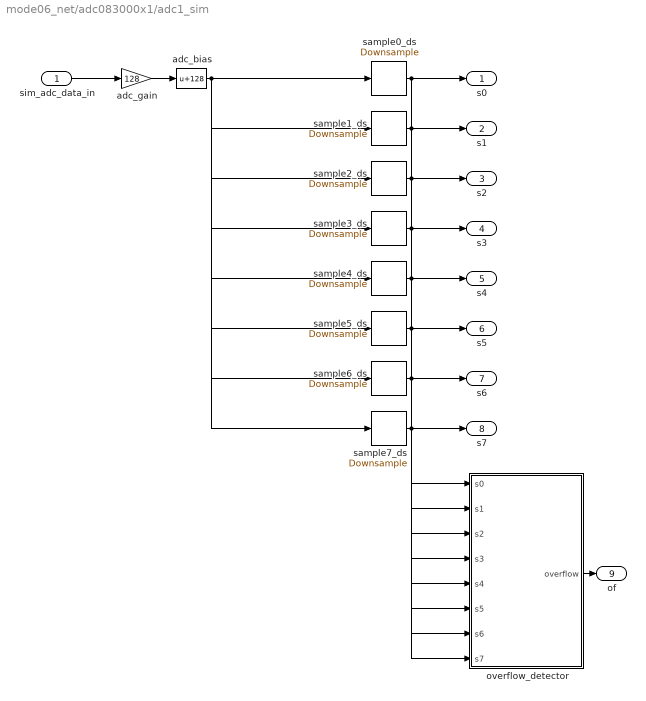
== system mode06_net/adc083000x1/adc1_sim ==
  sim_adc_data_in : Inport  OutDataType=sfix(16)  OutScaling=2^0
  adc_bias : Bias  Bias=128  SaturateOnIntegerOverflow=on
  adc_gain : Gain  Gain=128  ParameterDataType=sfix(16)  ParameterScaling=2^0  OutDataType=sfix(16)  OutScaling=2^0
  overflow_detector : Subsystem  AncestorBlock=casper_library/Misc/of_detect_bus  mask(of_detect_bus){nStreams=8, bit_width=8}
      mask prompts: nStreams "Number of Streams"; bit_width "Bit Width"
      mask init:
      | adc_overflow_detector_init(gcb, ...
      |     'nStreams', nStreams, ...
      |     'bit_width', bit_width);
  sample0_ds : dspsigops/Downsample  N=8  phase=1  ic=0  smode=Force single rate  fmode=Maintain input frame size
  sample1_ds : dspsigops/Downsample  N=8  phase=2  ic=0  smode=Force single rate  fmode=Maintain input frame size
  sample2_ds : dspsigops/Downsample  N=8  phase=3  ic=0  smode=Force single rate  fmode=Maintain input frame size
  sample3_ds : dspsigops/Downsample  N=8  phase=4  ic=0  smode=Force single rate  fmode=Maintain input frame size
  sample4_ds : dspsigops/Downsample  N=8  phase=5  ic=0  smode=Force single rate  fmode=Maintain input frame size
  sample5_ds : dspsigops/Downsample  N=8  phase=6  ic=0  smode=Force single rate  fmode=Maintain input frame size
  sample6_ds : dspsigops/Downsample  N=8  phase=7  ic=0  smode=Force single rate  fmode=Maintain input frame size
  sample7_ds : dspsigops/Downsample  N=8  phase=0  ic=0  smode=Force single rate  fmode=Maintain input frame size
  s0 : Outport  OutDataType=sfix(16)  OutScaling=2^0
  s1 : Outport  Port=2  OutDataType=sfix(16)  OutScaling=2^0
  s2 : Outport  Port=3  OutDataType=sfix(16)  OutScaling=2^0
  s3 : Outport  Port=4  OutDataType=sfix(16)  OutScaling=2^0
  s4 : Outport  Port=5  OutDataType=sfix(16)  OutScaling=2^0
  s5 : Outport  Port=6  OutDataType=sfix(16)  OutScaling=2^0
  s6 : Outport  Port=7  OutDataType=sfix(16)  OutScaling=2^0
  s7 : Outport  Port=8  OutDataType=sfix(16)  OutScaling=2^0
  of : Outport  Port=9  OutDataType=sfix(16)  OutScaling=2^0
  wires:
  sim_adc_data_in/1 -> adc_gain/1
  adc_gain/1 -> adc_bias/1
  overflow_detector/1(overflow) -> of/1
  adc_bias/1 -> sample0_ds/1, sample1_ds/1, sample2_ds/1, sample3_ds/1, sample4_ds/1, sample5_ds/1, sample6_ds/1, sample7_ds/1
  sample0_ds/1 -> overflow_detector/1(s0), s0/1
  sample1_ds/1 -> overflow_detector/2(s1), s1/1
  sample2_ds/1 -> overflow_detector/3(s2), s2/1
  sample3_ds/1 -> overflow_detector/4(s3), s3/1
  sample4_ds/1 -> overflow_detector/5(s4), s4/1
  sample5_ds/1 -> overflow_detector/6(s5), s5/1
  sample6_ds/1 -> overflow_detector/7(s6), s6/1
  sample7_ds/1 -> overflow_detector/8(s7), s7/1

== system mode06_net/arm/delay_pipe ==
  d : Inport
  q : Outport
  wires:
  d/1 -> q/1

== system mode06_net/cnt_rst/delay_pipe ==
  d : Inport
  q : Outport
  wires:
  d/1 -> q/1

== system mode06_net/dest_ip/delay_pipe ==
  d : Inport
  q : Outport
  wires:
  d/1 -> q/1

== system mode06_net/dest_port/delay_pipe ==
  d : Inport
  q : Outport
  wires:
  d/1 -> q/1

== system mode06_net/eth_rst/delay_pipe ==
  d : Inport
  q : Outport
  wires:
  d/1 -> q/1

== system mode06_net/ip_select/delay_pipe ==
  d : Inport
  q : Outport
  wires:
  d/1 -> q/1

== system mode06_net/port_select/delay_pipe ==
  d : Inport
  q : Outport
  wires:
  d/1 -> q/1

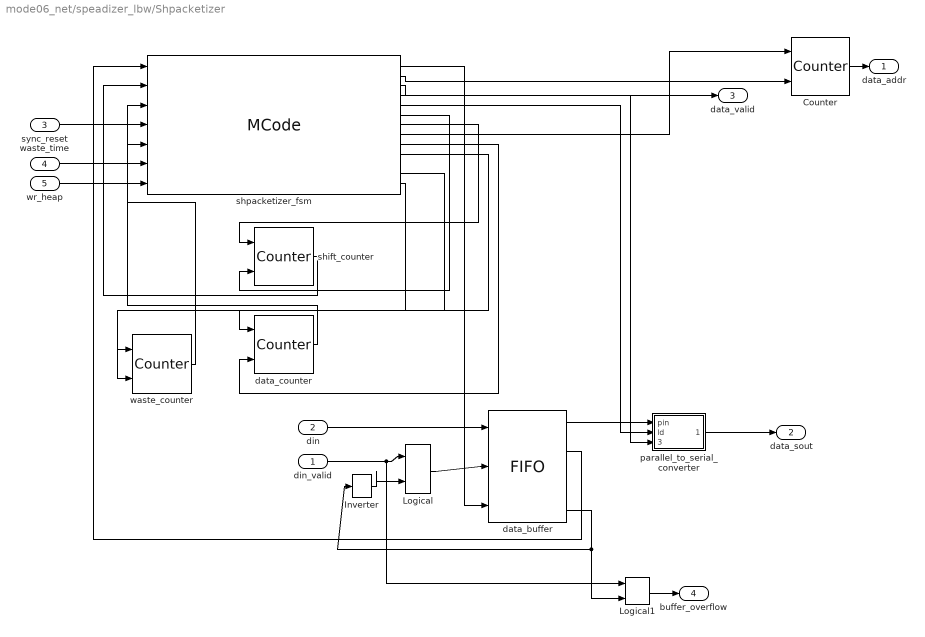
== system mode06_net/speadizer_lbw/Shpacketizer ==
  din_valid : Inport
  din : Inport  Port=2
  sync_reset : Inport  Port=3
  waste_time : Inport  Port=4
  wr_heap : Inport  Port=5
  Counter : xbsIndex_r4/Counter  cnt_type=Free Running  cnt_to=Inf  operation=Up  start_count=0  cnt_by_val=1  arith_type=Unsigned  n_bits=11  bin_pt=0  load_pin=off  rst=on  en=on  explicit_period=on  period=1  dbl_ovrd=off  use_behavioral_HDL=off  implementation=Fabric  use_rpm=off  block_type=counter
  Inverter : xbsIndex_r4/Inverter  en=off  latency=0  dbl_ovrd=off  block_type=inv
  Logical : xbsIndex_r4/Logical  logical_function=AND  inputs=2  en=off  latency=0  precision=Full  arith_type=Unsigned  n_bits=16  bin_pt=0  align_bp=on  dbl_ovrd=off  block_type=logical
  Logical1 : xbsIndex_r4/Logical  logical_function=AND  inputs=2  en=off  latency=0  precision=Full  arith_type=Unsigned  n_bits=16  bin_pt=0  align_bp=on  dbl_ovrd=off  block_type=logical
  data_buffer : xbsIndex_r4/FIFO  depth=128  percent_nbits=1  rst=off  en=off  use_dcount=off  use_almost_empty=off  almost_empty_thresh=2  use_almost_full=off  almost_full_thresh=14  dbl_ovrd=off  mem_type=Block RAM  explicit_period=off  block_type=fifo
      settings: block_version=10.1.3
  data_counter : xbsIndex_r4/Counter  cnt_type=Free Running  cnt_to=Inf  operation=Up  start_count=0  cnt_by_val=1  arith_type=Unsigned  n_bits=12  bin_pt=0  load_pin=off  rst=on  en=on  explicit_period=on  period=1  dbl_ovrd=off  use_behavioral_HDL=off  implementation=Fabric  use_rpm=off  block_type=counter
  parallel_to_serial_converter : Subsystem  AncestorBlock=casper_library/Flow_Control/parallel_to_serial_converter  mask(parallel_to_serial_converter){pin_width=128, sout_width=64}
      mask prompts: pin_width "Parallel Input Width"; sout_width "Serial Output Width"
      mask help:
      | This block takes as input a parallel bus of specified width.
      | When the load signal 'ld' is asserted, this data is broken into
      | pieces of width specified by the serial output width and
      | stored into different registers chained to form a shift register.
      | If the 'shift' input is subsequently asserted, the shift register
      | returns as output a new piece of data of width sout_width.  This data
      | is the next least significant piece of the original bus.  The converter
      | serializes SMALL ENDIAN.
      |
      | Note that the load operation automatically loads the least significant
      | bits into the register closest to the output, so the first 'shift'
      | assertion changes the data output from bits [sout_width-1:0] to
      | bits [2*sout_width-1:sout_width].
      mask init:
      | parallel_to_serial_converter_init(gcb, ...
      |     'pin_width', pin_width, ...
      |     'sout_width', sout_width);
  shift_counter : xbsIndex_r4/Counter  cnt_type=Free Running  cnt_to=Inf  operation=Up  start_count=0  cnt_by_val=1  arith_type=Unsigned  n_bits=1  bin_pt=0  load_pin=off  rst=on  en=on  explicit_period=on  period=1  dbl_ovrd=off  use_behavioral_HDL=off  implementation=Fabric  use_rpm=off  block_type=counter
  shpacketizer_fsm : xbsIndex_r4/MCode  mfname=shpacketizer_fsm  explicit_period=off  period=1  inputsTable={'boundInpExpr'=>['','','3','','31','','','',''],'inputs'=>['fifo_empty','shift_count','data_per_word','data_count','n_words','sync_reset','waste_count','waste_time','wr_heap']}  outputsTable={'outputs'=>['fifo_re','bram_addr_en','bram_we','serializer_shift','serializer_ld','shift_count_en','shift_count_rst','bram_addr_rst','data_count_en','data_count_rst','done','waste_count_en','waste_count_rst'],'suppressOut'=>['off','off','off','off','off','off','off','off','off','off','off','off','off']}  dbl_ovrd=off  enable_stdout=off  enable_debug=off  suppress_output=on  defparams={'data_per_word',1, 'n_words', 2047 }  hide_port_list={}  block_type=mcode
      settings: block_version=11.4
  waste_counter : xbsIndex_r4/Counter  cnt_type=Free Running  cnt_to=Inf  operation=Up  start_count=0  cnt_by_val=1  arith_type=Unsigned  n_bits=5  bin_pt=0  load_pin=off  rst=on  en=on  explicit_period=on  period=1  dbl_ovrd=off  use_behavioral_HDL=off  implementation=Fabric  use_rpm=off  block_type=counter
  data_addr : Outport
  data_sout : Outport  Port=2
  data_valid : Outport  Port=3
  buffer_overflow : Outport  Port=4
  wires:
  shpacketizer_fsm/13 -> waste_counter/1
  shpacketizer_fsm/12 -> waste_counter/2
  shpacketizer_fsm/10 -> data_counter/1
  shpacketizer_fsm/9 -> data_counter/2
  shpacketizer_fsm/8 -> Counter/1
  shpacketizer_fsm/2 -> Counter/2
  Counter/1 -> data_addr/1
  data_buffer/2 -> shpacketizer_fsm/1
  shpacketizer_fsm/7 -> shift_counter/1
  shift_counter/1 -> shpacketizer_fsm/2
  shpacketizer_fsm/6 -> shift_counter/2
  parallel_to_serial_converter/1(sout) -> data_sout/1
  din/1 -> data_buffer/1
  shpacketizer_fsm/3 -> data_valid/1
  shpacketizer_fsm/5 -> parallel_to_serial_converter/2(ld)
  shpacketizer_fsm/4 -> parallel_to_serial_converter/3(shift)
  shpacketizer_fsm/1 -> data_buffer/3
  data_buffer/1 -> parallel_to_serial_converter/1(pin)
  Logical/1 -> data_buffer/2
  din_valid/1 -> Logical/1, Logical1/1
  Inverter/1 -> Logical/2
  data_buffer/4 -> Inverter/1, Logical1/2
  Logical1/1 -> buffer_overflow/1
  wr_heap/1 -> shpacketizer_fsm/7
  waste_time/1 -> shpacketizer_fsm/6
  data_counter/1 -> shpacketizer_fsm/3
  sync_reset/1 -> shpacketizer_fsm/4
  waste_counter/1 -> shpacketizer_fsm/5

== system mode06_net/sync_en/delay_pipe ==
  d : Inport
  q : Outport
  wires:
  d/1 -> q/1

== system mode06_net/sync_period/delay_pipe ==
  d : Inport
  q : Outport
  wires:
  d/1 -> q/1

== system mode06_net/sync_sel/delay_pipe ==
  d : Inport
  q : Outport
  wires:
  d/1 -> q/1

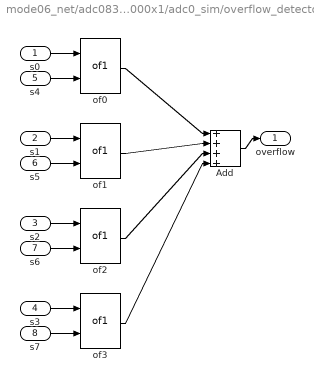
== system mode06_net/adc083000x1/adc0_sim/overflow_detector ==
  s0 : Inport  OutDataType=fixdt(1, 16)  OutScaling=2^0
  s1 : Inport  Port=2  OutDataType=fixdt(1, 16)  OutScaling=2^0
  s2 : Inport  Port=3  OutDataType=fixdt(1, 16)  OutScaling=2^0
  s3 : Inport  Port=4  OutDataType=fixdt(1, 16)  OutScaling=2^0
  s4 : Inport  Port=5  OutDataType=fixdt(1, 16)  OutScaling=2^0
  s5 : Inport  Port=6  OutDataType=fixdt(1, 16)  OutScaling=2^0
  s6 : Inport  Port=7  OutDataType=fixdt(1, 16)  OutScaling=2^0
  s7 : Inport  Port=8  OutDataType=fixdt(1, 16)  OutScaling=2^0
  Add : Sum  Inputs=++++  OutDataType=fixdt(1, 16)  OutScaling=2^-10
  of{0..3} (4 alike) : casper_library_misc/of1  SystemSampleTime=-1  bit_num=0  n_adc_bits=8
  overflow : Outport  OutDataType=fixdt(1, 16)  OutScaling=2^0
  wires:
  s0/1 -> of0/1
  s4/1 -> of0/2
  of0/1 -> Add/1
  s1/1 -> of1/1
  s5/1 -> of1/2
  of1/1 -> Add/2
  s2/1 -> of2/1
  s6/1 -> of2/2
  of2/1 -> Add/3
  s3/1 -> of3/1
  s7/1 -> of3/2
  of3/1 -> Add/4
  Add/1 -> overflow/1

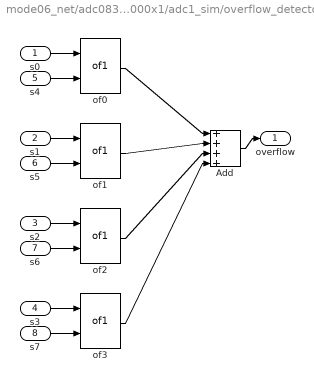
== system mode06_net/adc083000x1/adc1_sim/overflow_detector ==
  s0 : Inport  OutDataType=fixdt(1, 16)  OutScaling=2^0
  s1 : Inport  Port=2  OutDataType=fixdt(1, 16)  OutScaling=2^0
  s2 : Inport  Port=3  OutDataType=fixdt(1, 16)  OutScaling=2^0
  s3 : Inport  Port=4  OutDataType=fixdt(1, 16)  OutScaling=2^0
  s4 : Inport  Port=5  OutDataType=fixdt(1, 16)  OutScaling=2^0
  s5 : Inport  Port=6  OutDataType=fixdt(1, 16)  OutScaling=2^0
  s6 : Inport  Port=7  OutDataType=fixdt(1, 16)  OutScaling=2^0
  s7 : Inport  Port=8  OutDataType=fixdt(1, 16)  OutScaling=2^0
  Add : Sum  Inputs=++++  OutDataType=fixdt(1, 16)  OutScaling=2^-10
  of{0..3} (4 alike) : casper_library_misc/of1  SystemSampleTime=-1  bit_num=0  n_adc_bits=8
  overflow : Outport  OutDataType=fixdt(1, 16)  OutScaling=2^0
  wires:
  s0/1 -> of0/1
  s4/1 -> of0/2
  of0/1 -> Add/1
  s1/1 -> of1/1
  s5/1 -> of1/2
  of1/1 -> Add/2
  s2/1 -> of2/1
  s6/1 -> of2/2
  of2/1 -> Add/3
  s3/1 -> of3/1
  s7/1 -> of3/2
  of3/1 -> Add/4
  Add/1 -> overflow/1

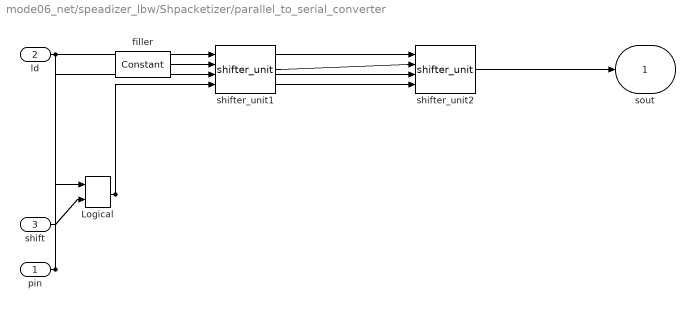
== system mode06_net/speadizer_lbw/Shpacketizer/parallel_to_serial_converter ==
  pin : Inport
  ld : Inport  Port=2
  shift : Inport  Port=3
  Logical : xbsIndex_r4/Logical  logical_function=OR  inputs=2  en=off  latency=0  precision=Full  arith_type=Unsigned  n_bits=16  bin_pt=0  align_bp=on  dbl_ovrd=off  block_type=logical
  filler : xbsIndex_r4/Constant  arith_type=Unsigned  const=0  n_bits=sout_width  bin_pt=0  explicit_period=on  period=1  equ=P=C  opselect=C  inp2=PCIN>>17  opr=+  inp1=P  carry=CIN  dbl_ovrd=off  block_type=constant
  shifter_unit1 : casper_library_flow_control/shifter_unit  SystemSampleTime=-1  data_width=64  pin_offset=0
  shifter_unit2 : casper_library_flow_control/shifter_unit  SystemSampleTime=-1  data_width=64  pin_offset=64
  sout : Outport  OutDataType=sfix(16)  OutScaling=2^0
  wires:
  ld/1 -> Logical/1, shifter_unit1/1, shifter_unit2/1
  shift/1 -> Logical/2
  filler/1 -> shifter_unit1/2
  pin/1 -> shifter_unit1/3, shifter_unit2/3
  Logical/1 -> shifter_unit1/4, shifter_unit2/4
  shifter_unit1/1 -> shifter_unit2/2
  shifter_unit2/1 -> sout/1
